simulink model "FOFDM"  (Simulink 8.5)
settings: Solver=FixedStepDiscrete  StartTime=0.0  StopTime=1.0  FixedStep=1e-8  MaxStep=1/40e6  RelTol=1/40e6
model workspace (MAT data in the model file):
  M = Simulink.Parameter
  M.Value = 16
  M.DataType = 'auto'
  N = Simulink.Parameter
  N.Value = 48
  N.DataType = 'auto'
  C = Simulink.Parameter
  C.Value = 16
  C.DataType = 'auto'
  sampleTime = Simulink.Parameter
  sampleTime.Value = 8e-06
  sampleTime.DataType = 'auto'
libraries: dspxfrm3 x2, dspindex x2, dsparch4 x2, commdigbbndam3 x2, commchan3 x1, commrandsrc2 x1, commsink2 x1, commutil2 x1, dspobslib x1, dspsigops x1
settings Model: Creator=levyg  LastModifiedBy=levyg
settings DataIOCC: SignalLoggingSaveFormat=Dataset
settings OptimizationCC: ExpressionDepthLimit=128
settings DebuggingCC: UnderspecifiedInitializationDetection=Simplified  MergeDetectMultiDrivingBlocksExec=error  FcnCallInpInsideContextMsg=EnableAllAsError  StateNameClashWarn=none
settings GRTTargetCC: CombineOutputUpdateFcns=on  GRTInterface=off

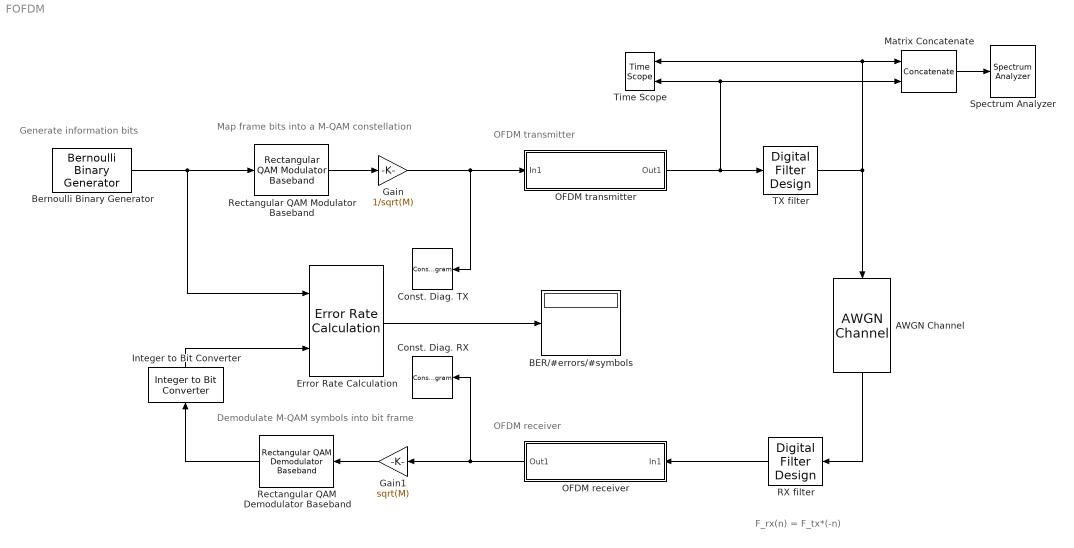
== system FOFDM ==
  note: F_rx(n) = F_tx*(-n)
  note: OFDM transmitter
  note: Map frame bits into a M-QAM constellation
  note: Generate information bits
  note: OFDM receiver
  note: Demodulate M-QAM symbols into bit frame
  AWGN Channel : commchan3/AWGN Channel  InputProcessing=Columns as channels (frame based)  seed=67  noiseMode="Signal to noise ratio  (Eb/No)"  EbNodB=35  EsNodB=10  SNRdB=10  bitsPerSym=N*log2(M)  Ps=1  Tsym=sampleTime  variance=1
  BER/#errors/#symbols : Display
  Bernoulli Binary Generator : commrandsrc2/Bernoulli Binary Generator  P=0.5  seed=20394875  Ts=1/(N*log2(M))*sampleTime  frameBased=on  sampPerFrame=N*log2(M)  orient=off  outDataType=boolean
  Const. Diag. RX : ConstellationDiagram
  Const. Diag. TX : ConstellationDiagram
  Error Rate Calculation : commsink2/Error Rate Calculation  N=0  st_delay=0  cp_mode=Entire frame  subframe=[]  PMode=Port  WsName=ErrorVec  RsMode2=off  stop=off  numErr=100  maxBits=1e6
  Gain : Gain  Gain=1/sqrt(M)
  Gain1 : Gain  Gain=sqrt(M)
  Integer to Bit Converter : commutil2/Integer to Bit Converter  nbits=log2(M)  signedInputValues=Unsigned  bitOrder=MSB first  outDtype=Inherit via internal rule
  Matrix Concatenate : Concatenate  Mode=Multidimensional array  ConcatenateDimension=2
  OFDM receiver : Subsystem
  OFDM transmitter : Subsystem
  RX filter : dsparch4/Digital Filter Design  mwdsp_browser_bugfix_var=off
  Rectangular QAM Demodulator Baseband : commdigbbndam3/Rectangular QAM Demodulator Baseband  M=M  PowType=Min. distance between symbols  MinDist=2  AvgPow=1  PeakPow=1  Ph=0  Dec=Gray  Mapping=[0:15]  OutType=Integer  DecType=Hard decision  VarSource=Dialog  Variance=1  outDtype1=Inherit via internal rule  outDtype2=Inherit via internal rule  derotateFactorDTMode=Specify word length  derotateFactorWordLen=16  denormFactorWordLen=16  prodOutWordLen=32  prodOutRoundingMode=Floor  prodOutOverflowMode=Wrap  sumWordLen=32
  Rectangular QAM Modulator Baseband : commdigbbndam3/Rectangular QAM Modulator Baseband  M=M  InType=Bit  Enc=Gray  Mapping=[0:15]  PowType=Min. distance between symbols  MinDist=2  AvgPow=1  PeakPow=1  Ph=0  outDtype=double  outWordLen=16  outUDDataType=sfix(16)  outFracLenMode=Best precision  outFracLen=15
  Spectrum Analyzer : SpectrumAnalyzer
  TX filter : dsparch4/Digital Filter Design  mwdsp_browser_bugfix_var=off
  Time Scope : TimeScope  DefaultConfigurationName=spbscopes.TimeScopeBlockCfg  NumInputPorts=2
  wires:
  Rectangular QAM Modulator Baseband/1 -> Gain/1
  Gain/1 -> Const. Diag. TX/1, OFDM transmitter/1(In1)
  OFDM receiver/1(Out1) -> Const. Diag. RX/1, Gain1/1
  Gain1/1 -> Rectangular QAM Demodulator Baseband/1
  Error Rate Calculation/1 -> BER/#errors/#symbols/1
  Rectangular QAM Demodulator Baseband/1 -> Integer to Bit Converter/1
  Integer to Bit Converter/1 -> Error Rate Calculation/2
  AWGN Channel/1 -> RX filter/1
  Bernoulli Binary Generator/1 -> Error Rate Calculation/1, Rectangular QAM Modulator Baseband/1
  TX filter/1 -> Matrix Concatenate/1, Time Scope/1, AWGN Channel/1
  OFDM transmitter/1(Out1) -> Matrix Concatenate/2, Time Scope/2, TX filter/1
  RX filter/1 -> OFDM receiver/1(In1)
  Matrix Concatenate/1 -> Spectrum Analyzer/1

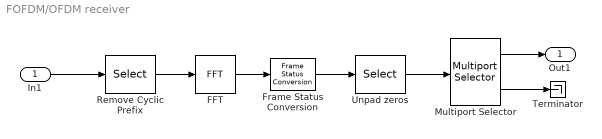
== system FOFDM/OFDM receiver ==
  In1 : Inport
  FFT : dspxfrm3/FFT  CompMethod=Table lookup  TableOpt=NEW  TableOptActive=Speed  BitRevOrder=off  InheritFFTLength=on  FFTLength=64  WrapInput=on  RowConvenienceOn=on  FFTImplementation=Auto  SkipNorm=off  firstCoeffDataTypeStr=Inherit: Same word length as input  firstCoeffLastDataTypeStr=Inherit: Same word length as input  outputMin=[]  outputMax=[]  roundingMode=Floor  overflowMode=off
  Frame Status Conversion : dspobslib/Frame Status Conversion  growRefPort=off  outframe=Frame-based
  Multiport Selector : dspindex/Multiport Selector  rowsOrCols=Rows  idxCellArray={[1:5 7:19 21:26 28:33 35:47 49:53], [6 20 34 48]}  idxErrMode=Clip Index
  Remove Cyclic Prefix : Selector  NumberOfDimensions=2  InputPortWidth=2^(ceil(log2(N)))  IndexOptions=Index vector (dialog),Select all  Indices=[C+1:80],1  OutputSizes=[(-2)],1
  Terminator : Terminator
  Unpad zeros : Selector  NumberOfDimensions=2  InputPortWidth=2^(ceil(log2(N)))  IndexOptions=Index vector (dialog),Select all  Indices=[39:64 1:27],1  OutputSizes=[(-2)],1
  Out1 : Outport
  wires:
  Multiport Selector/1 -> Out1/1
  In1/1 -> Remove Cyclic Prefix/1
  Remove Cyclic Prefix/1 -> FFT/1
  FFT/1 -> Frame Status Conversion/1
  Frame Status Conversion/1 -> Unpad zeros/1
  Unpad zeros/1 -> Multiport Selector/1
  Multiport Selector/2 -> Terminator/1

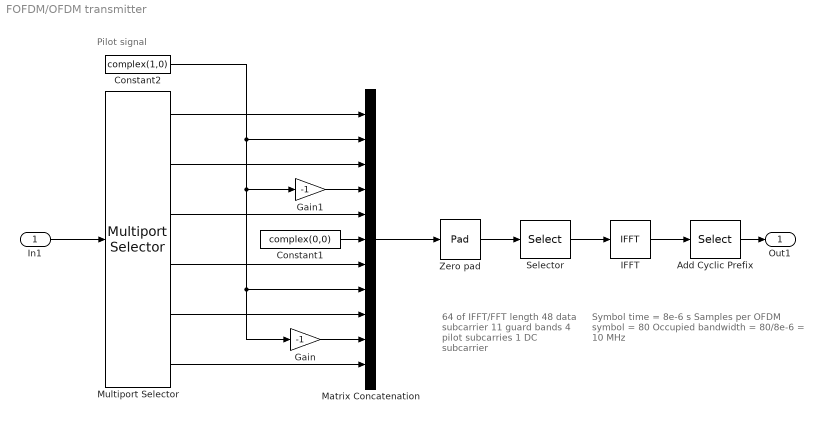
== system FOFDM/OFDM transmitter ==
  note: Symbol time = 8e-6 s
      | Samples per OFDM symbol = 80
      | Occupied bandwidth = 80/8e-6 = 10 MHz
  note: 64 of IFFT/FFT length
      | 48 data subcarrier
      | 11 guard bands
      | 4 pilot subcarries
      | 1 DC subcarrier
  note: Pilot signal
  In1 : Inport
  Add Cyclic Prefix : Selector  NumberOfDimensions=2  InputPortWidth=2^(ceil(log2(N)))  IndexOptions=Index vector (dialog),Select all  Indices=[2^(ceil(log2(N)))-C+1:2^(ceil(log2(N))) 1:2^(ceil(log2(N)))],1  OutputSizes=[(-2)],1
  Constant1 : Constant  Value=complex(0,0)  SampleTime=sampleTime
  Constant2 : Constant  Value=complex(1,0)  SampleTime=sampleTime
  Gain : Gain  Gain=-1
  Gain1 : Gain  Gain=-1
  IFFT : dspxfrm3/IFFT  CompMethod=Table lookup  TableOpt=NEW  TableOptActive=Speed  BitRevOrder=off  cs_in=off  SkipNorm=on  InheritFFTLength=on  FFTLength=64  WrapInput=on  mode=Complex  outSamplingMode=Sample based  RowConvenienceOn=on  FFTImplementation=Auto  firstCoeffDataTypeStr=Inherit: Same word length as input  firstCoeffLastDataTypeStr=Inherit: Same word length as input  outputMin=[]  outputMax=[]  roundingMode=Floor  overflowMode=off
  Matrix Concatenation : Concatenate  NumInputs=11  Mode=Multidimensional array
  Multiport Selector : dspindex/Multiport Selector  rowsOrCols=Rows  idxCellArray={1:5, 6:18, 19:24, 25:30, 31:43, 44:48}  idxErrMode=Clip Index
  Selector : Selector  NumberOfDimensions=2  InputPortWidth=3  IndexOptions=Index vector (dialog),Select all  Indices=[27:64 1:26],1  OutputSizes=1,1
  Zero pad : dspsigops/Pad  padAlong=Columns  dimsToPad=1  valSrc=Specify via dialog  padVal=0  spec=Output size  padNumOutRowsSpecMethod=User-specified  numOutRows=64  padNumOutColsSpecMethod=User-specified  numOutCols=1  isVarDimsMode=off  padBeginning=0  padEnd=0  outSizeMode=User-specified  outSize=1  padSigAt=End  trunc_flag=None  roundingMode=Floor  overflowMode=off  truncOrWrapMode=Truncate  wrap_flag=None
  Out1 : Outport
  wires:
  In1/1 -> Multiport Selector/1
  Multiport Selector/1 -> Matrix Concatenation/1
  Multiport Selector/2 -> Matrix Concatenation/3
  Multiport Selector/3 -> Matrix Concatenation/5
  Multiport Selector/6 -> Matrix Concatenation/11
  Multiport Selector/5 -> Matrix Concatenation/9
  Multiport Selector/4 -> Matrix Concatenation/7
  Constant1/1 -> Matrix Concatenation/6
  Constant2/1 -> Matrix Concatenation/2, Gain1/1, Gain/1, Matrix Concatenation/8
  Gain/1 -> Matrix Concatenation/10
  Matrix Concatenation/1 -> Zero pad/1
  Zero pad/1 -> Selector/1
  Selector/1 -> IFFT/1
  IFFT/1 -> Add Cyclic Prefix/1
  Add Cyclic Prefix/1 -> Out1/1
  Gain1/1 -> Matrix Concatenation/4
